simulink model "deadlock"  (Simulink 10.0)
settings: Solver=ode45  StartTime=0.0  StopTime=10  FixedStep=1  MaxStep=inf  RelTol=1e-3  EnableMultiTasking=on
InitFcn:
  | EXT_PACKET = 1;
  | ACK_PACKET = 2;
  | RX = 1;
  | TX = 2;
  | COMMS_DELAY = 1;
libraries: simeventsgenerators1 x8, simeventsserver1 x8, simeventsattributes2 x6, simeventssink1 x4, simeventsgates1 x2, simeventsqueue1 x2, simeventsrouting1 x2, simeventstranslate1 x2, simulink x1
settings Model: Creator=The MathWorks Inc.  LastModifiedBy=bhisma
settings DataIOCC: LimitDataPoints=on  SignalLoggingSaveFormat=ModelDataLogs  SaveOutput=off  SaveTime=off
settings OptimizationCC: ExpressionDepthLimit=2147483647  EfficientMapNaN2IntZero=off
settings DebuggingCC: ReadBeforeWriteMsg=DisableAll  WriteAfterWriteMsg=DisableAll  WriteAfterReadMsg=DisableAll  AlgebraicLoopMsg=error  FcnCallInpInsideContextMsg=warning  StateNameClashWarn=warning
settings SFSimCC: SimParseCustomCode=off
settings GRTTargetCC: GeneratePreprocessorConditionals=Disable all
settings ConfigComp: CovExternalEMLEnable=off
settings SimEventsCC: propDiagAttribOutput=1  propDiagFcnCallOutput=1  propDiagStatOutput=0  propPreventDuplicateEvents=0

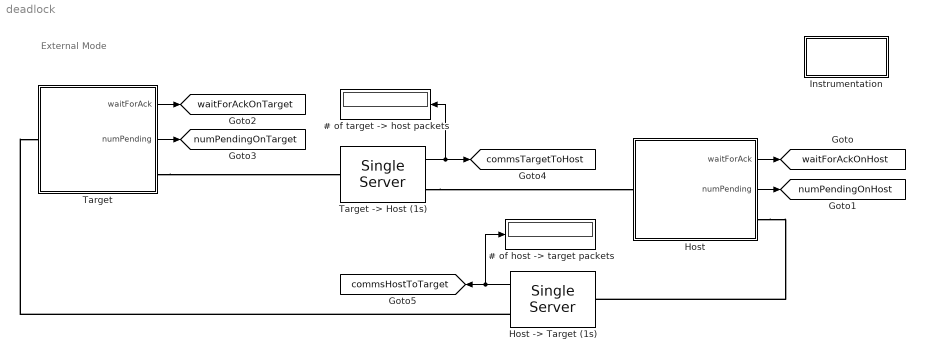
== system deadlock ==
  note: External Mode
  "# of host -> target packets" : Display
  "# of target -> host packets" : Display
  Host : Subsystem
  "Host -> Target (1s)" : simeventsserver1/Single Server  Priority=1  SystemSampleTime=-1  ServiceTimeFrom=Dialog  ServiceTime=COMMS_DELAY  AttributeName=ServiceTime  PriorityServiceCompletion=1  PermitPreemption=off  SortingAttributeName=PriorityAttributeName  SortingDirection=Ascending  WriteToAttribute=off  ResidualAttributeName=ResidualServiceTime  CreateAttribute=on  EnableTOPort=off  StatNumberDeparted=On  StatNumberInBlock=Off  StatNumberPreempted=Off  StatPendingEntity=Off  StatAverageWait=Off  StatUtilization=Off  StatNumberTimedout=Off
  Instrumentation : Subsystem
      settings: RequestExecContextInheritance=on
      mask Display: disp('Scopes');
  Target : Subsystem
  "Target -> Host (1s)" : simeventsserver1/Single Server  Priority=1  SystemSampleTime=-1  ServiceTimeFrom=Dialog  ServiceTime=COMMS_DELAY  AttributeName=ServiceTime  PriorityServiceCompletion=1  PermitPreemption=off  SortingAttributeName=PriorityAttributeName  SortingDirection=Ascending  WriteToAttribute=off  ResidualAttributeName=ResidualServiceTime  CreateAttribute=on  EnableTOPort=off  StatNumberDeparted=On  StatNumberInBlock=Off  StatNumberPreempted=Off  StatPendingEntity=Off  StatAverageWait=Off  StatUtilization=Off  StatNumberTimedout=Off
  tag scope: commsHostToTarget=global, commsTargetToHost=global, numPendingOnHost=global, numPendingOnTarget=global, waitForAckOnHost=global, waitForAckOnTarget=global
  wires:
  Host/1(waitForAck) -> [waitForAckOnHost]
  Host/2(numPending) -> [numPendingOnHost]
  Target/1(waitForAck) -> [waitForAckOnTarget]
  Target/2(numPending) -> [numPendingOnTarget]
  "Target -> Host (1s)"/1 -> [commsTargetToHost], "# of target -> host packets"/1
  "Host -> Target (1s)"/1 -> [commsHostToTarget], "# of host -> target packets"/1
  connections:
  Target/RConn1 -- "Target -> Host (1s)"/LConn1
  "Target -> Host (1s)"/RConn1 -- Host/LConn1
  Host/RConn1 -- "Host -> Target (1s)"/LConn1
  "Host -> Target (1s)"/RConn1 -- Target/LConn1

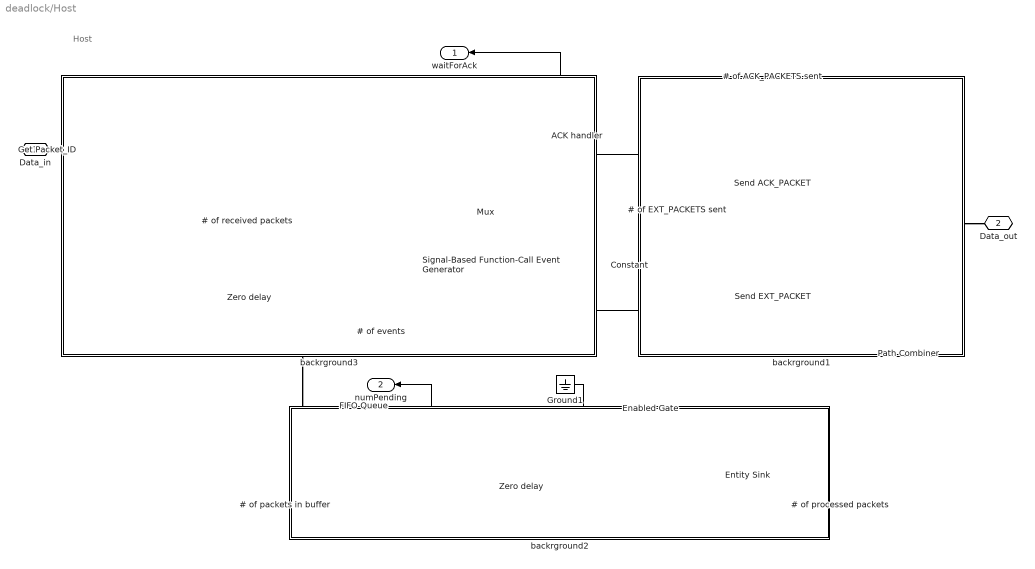
== system deadlock/Host ==
  note: Host
  # of ACK_PACKETS sent : Display
  # of EXT_PACKETS sent : Display
  # of events : Display
  # of packets in buffer : Display
  # of processed packets : Display
  # of received packets : Display
  ACK handler : Stateflow chart  TreatAsAtomicUnit=on
      settings: PropExecContextOutsideSubsystem=on
  Constant : Constant
  Enabled Gate : simeventsgates1/Enabled Gate  Priority=1  SystemSampleTime=-1  SpecifyEventPriority=off  PriorityGateEnableOpenClose=2000  StatNumberDeparted=Off
  Entity Sink : simeventssink1/Entity Sink  Priority=1  SystemSampleTime=-1  AvailableForArrivals=on  StatNumberArrived=On
  FIFO Queue : simeventsqueue1/FIFO Queue  Priority=1  SystemSampleTime=-1  Capacity=2  EnableTOPort=off  StatNumberDeparted=Off  StatNumberInBlock=On  StatPendingEntity=Off  StatAverageWait=Off  StatAverageQueueLength=Off  StatNumberTimedout=Off
      settings: AttributesFormatString=Capacity = %<Capacity>
  Get Packet_ID : simeventsattributes2/Get Attribute  Priority=1  SystemSampleTime=-1  AttributeName=PacketID  AttributeMissing=Error  AttributeDefaultValue=1  AttributeSendTiming=After entity departure  AttributeTreatAsVector=1  StatNumberDeparted=Off  EvaluatedDefaultAttributeValue={[]}
  Ground1 : Ground
  Mux : Mux  Inputs=2
  Path Combiner : simeventsrouting1/Path Combiner  Priority=1  SystemSampleTime=-1  NumberInputPorts=2  InputPortPrecedence=IN1 port  InitialSeed=45675  SpecifyEventPriority=off  PriorityPathCombinerPortPrecedenceSelection=4100  StatNumberDeparted=Off  StatLastArrivalPort=Off  EvaluatedNumPorts=2
  Send ACK_PACKET : Subsystem
  Send EXT_PACKET : Subsystem
  Signal-Based Function-Call Event Generator : simeventsgenerators1/Event Generators/Signal-Based Function-Call Event Generator  Priority=1  SystemSampleTime=-1  GenerateFunctionCallUpon=Change in signal from port vc  SignalEdgeOption=Either  EnableE1Port=off  EnableF2Port=off  EnableE2Port=off  SpecifyEventPriority=off  PriorityFunctionCall=200  FunctionCallDelayFrom=Dialog  DelayFunctionCall=0  StatNumberF1Calls=On  StatNumberF2Calls=Off  MaskBlockType=none
  Zero delay : simeventsserver1/Single Server  Priority=1  SystemSampleTime=-1  ServiceTimeFrom=Dialog  ServiceTime=0  AttributeName=ServiceTime  PriorityServiceCompletion=1  PermitPreemption=off  SortingAttributeName=PriorityAttributeName  SortingDirection=Ascending  WriteToAttribute=off  ResidualAttributeName=ResidualServiceTime  CreateAttribute=on  EnableTOPort=off  StatNumberDeparted=Off  StatNumberInBlock=Off  StatNumberPreempted=Off  StatPendingEntity=Off  StatAverageWait=Off  StatUtilization=Off  StatNumberTimedout=Off
  "Zero delay " : simeventsserver1/Single Server  Priority=1  SystemSampleTime=-1  ServiceTimeFrom=Dialog  ServiceTime=0  AttributeName=ServiceTime  PriorityServiceCompletion=1  PermitPreemption=off  SortingAttributeName=PriorityAttributeName  SortingDirection=Ascending  WriteToAttribute=off  ResidualAttributeName=ResidualServiceTime  CreateAttribute=on  EnableTOPort=off  StatNumberDeparted=On  StatNumberInBlock=On  StatNumberPreempted=Off  StatPendingEntity=Off  StatAverageWait=Off  StatUtilization=Off  StatNumberTimedout=Off
  backrground1 : Subsystem
      mask Display: disp('')
  backrground2 : Subsystem
      mask Display: disp('')
  backrground3 : Subsystem
      mask Display: disp('')
  Data_in : PMIOPort  Side=Left
  Data_out : PMIOPort  Port=2  Side=Right
  waitForAck : Outport
  numPending : Outport  Port=2
  wires:
  Entity Sink/1 -> # of processed packets/1
  Constant/1 -> Send EXT_PACKET/1(waitForAck)
  FIFO Queue/1 -> numPending/1, # of packets in buffer/1
  Get Packet_ID/1 -> ACK handler/1(pID)
  "Zero delay "/2 -> Signal-Based Function-Call Event Generator/1
  ACK handler/1(waitForAck) -> waitForAck/1
  Send ACK_PACKET/1(numAckPacketsSent) -> # of ACK_PACKETS sent/1
  Send EXT_PACKET/1(numExtPacketsSent) -> # of EXT_PACKETS sent/1
  Signal-Based Function-Call Event Generator/2 -> # of events/1
  Mux/1 -> ACK handler/Trigger
  Signal-Based Function-Call Event Generator/1 -> Mux/1
  ACK handler/2(sendAck()) -> Send ACK_PACKET/1(trig)
  Ground1/1 -> Enabled Gate/1
  Send EXT_PACKET/2(txExtPacket) -> Mux/2
  "Zero delay "/1 -> # of received packets/1
  connections:
  Enabled Gate/RConn1 -- Entity Sink/LConn1
  Path Combiner/RConn1 -- Data_out/RConn1
  Send ACK_PACKET/RConn1 -- Path Combiner/LConn1
  Send EXT_PACKET/RConn1 -- Path Combiner/LConn2
  FIFO Queue/RConn1 -- Zero delay/LConn1
  Zero delay/RConn1 -- Enabled Gate/LConn1
  Data_in/RConn1 -- Get Packet_ID/LConn1
  Get Packet_ID/RConn1 -- "Zero delay "/LConn1
  "Zero delay "/RConn1 -- FIFO Queue/LConn1

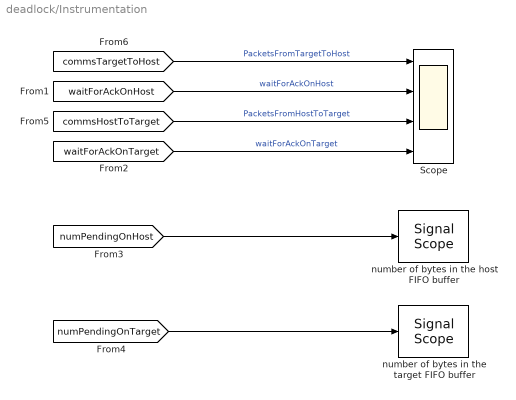
== system deadlock/Instrumentation ==
  Scope : Scope  NumInputPorts=4
  number of bytes in the host FIFO buffer : simeventssink1/Signal Scope  Priority=1  SystemSampleTime=-1  PlotType=Stair  InputType=Signal  NumInputs=1  AttributeNameY=Count  XInputOptionSignal=Event time  XInputOptionEntity=Event time  AttributeNameX=Count  EnableEntityOutport=on  XMin=0  XMax=10  XLimitExceededOption=Stretch axis limits  YLimitExceededOption=Stretch axis limits  AxisGrid=on  AxisLegend=off  LineDisables=""  LineColors=b  LineStyles=-  LineMarkers=.  OpenScopeAtSimStart=on  Title=Packets in host buffer  YLabel=#n  XLabel=Time  FigurePosition=[72 229 231 135]  AxisZoom=off  DataStoreOption=Limited  DataPointsLimit=10000  StatNumberArrived=Off  ShowCountPlotted=off  ShowToolbar=on
      settings: YMin=-1  YMax=3
  number of bytes in the target FIFO buffer : simeventssink1/Signal Scope  Priority=1  SystemSampleTime=-1  PlotType=Stair  InputType=Signal  NumInputs=1  AttributeNameY=Count  XInputOptionSignal=Event time  XInputOptionEntity=Event time  AttributeNameX=Count  EnableEntityOutport=on  XMin=0  XMax=10  XLimitExceededOption=Stretch axis limits  YLimitExceededOption=Stretch axis limits  AxisGrid=on  AxisLegend=off  LineDisables=""  LineColors=b  LineStyles=-  LineMarkers=.  OpenScopeAtSimStart=on  Title=Packets in target buffer  YLabel=#n  XLabel=Time  FigurePosition=[72 229 231 135]  AxisZoom=off  DataStoreOption=Limited  DataPointsLimit=10000  StatNumberArrived=Off  ShowCountPlotted=off  ShowToolbar=on
      settings: YMin=-1  YMax=3
  wires:
  [numPendingOnHost] -> number of bytes in the host FIFO buffer/1
  [numPendingOnTarget] -> number of bytes in the target FIFO buffer/1
  [commsTargetToHost] -> Scope/1  "PacketsFromTargetToHost"
  [waitForAckOnHost] -> Scope/2  "waitForAckOnHost"
  [commsHostToTarget] -> Scope/3  "PacketsFromHostToTarget"
  [waitForAckOnTarget] -> Scope/4  "waitForAckOnTarget"

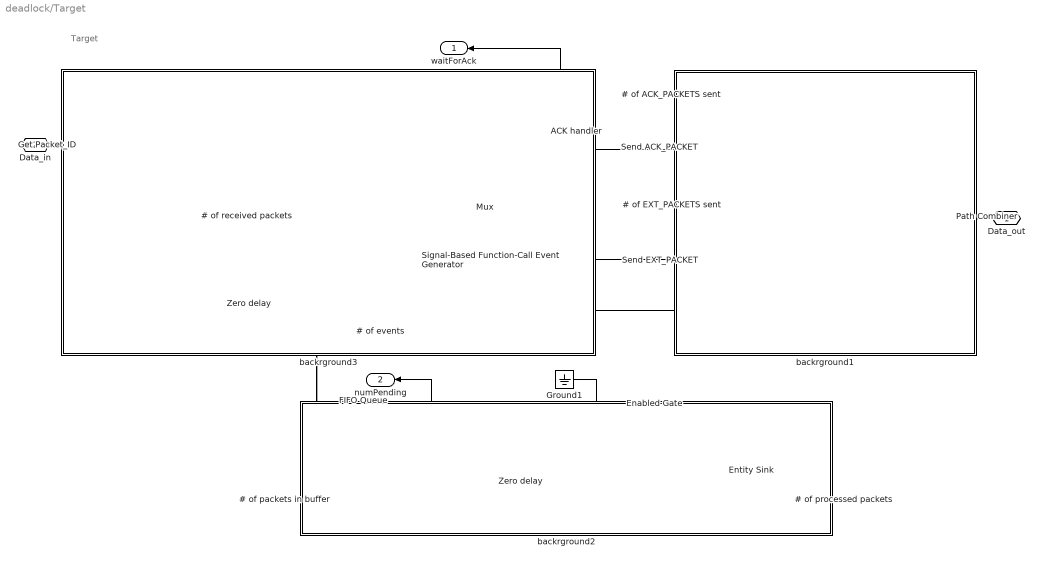
== system deadlock/Target ==
  note: Target
  # of ACK_PACKETS sent : Display
  # of EXT_PACKETS sent : Display
  # of events : Display
  # of packets in buffer : Display
  # of processed packets : Display
  # of received packets : Display
  ACK handler : Stateflow chart  TreatAsAtomicUnit=on
      settings: PropExecContextOutsideSubsystem=on
  Enabled Gate : simeventsgates1/Enabled Gate  Priority=1  SystemSampleTime=-1  SpecifyEventPriority=off  PriorityGateEnableOpenClose=2000  StatNumberDeparted=Off
  Entity Sink : simeventssink1/Entity Sink  Priority=1  SystemSampleTime=-1  AvailableForArrivals=on  StatNumberArrived=On
  FIFO Queue : simeventsqueue1/FIFO Queue  Priority=1  SystemSampleTime=-1  Capacity=2  EnableTOPort=off  StatNumberDeparted=Off  StatNumberInBlock=On  StatPendingEntity=Off  StatAverageWait=Off  StatAverageQueueLength=Off  StatNumberTimedout=Off
      settings: AttributesFormatString=Capacity = %<Capacity>
  Get Packet_ID : simeventsattributes2/Get Attribute  Priority=1  SystemSampleTime=-1  AttributeName=PacketID  AttributeMissing=Error  AttributeDefaultValue=1  AttributeSendTiming=After entity departure  AttributeTreatAsVector=1  StatNumberDeparted=Off  EvaluatedDefaultAttributeValue={[]}
  Ground1 : Ground
  Mux : Mux  Inputs=2
  Path Combiner : simeventsrouting1/Path Combiner  Priority=1  SystemSampleTime=-1  NumberInputPorts=2  InputPortPrecedence=IN1 port  InitialSeed=45675  SpecifyEventPriority=off  PriorityPathCombinerPortPrecedenceSelection=4100  StatNumberDeparted=Off  StatLastArrivalPort=Off  EvaluatedNumPorts=2
  Send ACK_PACKET : Subsystem
  Send EXT_PACKET : Subsystem
  Signal-Based Function-Call Event Generator : simeventsgenerators1/Event Generators/Signal-Based Function-Call Event Generator  Priority=1  SystemSampleTime=-1  GenerateFunctionCallUpon=Change in signal from port vc  SignalEdgeOption=Rising  EnableE1Port=off  EnableF2Port=off  EnableE2Port=off  SpecifyEventPriority=on  PriorityFunctionCall=2  FunctionCallDelayFrom=Dialog  DelayFunctionCall=0  StatNumberF1Calls=On  StatNumberF2Calls=Off  MaskBlockType=none
  Zero delay : simeventsserver1/Single Server  Priority=1  SystemSampleTime=-1  ServiceTimeFrom=Dialog  ServiceTime=0  AttributeName=ServiceTime  PriorityServiceCompletion=1  PermitPreemption=off  SortingAttributeName=PriorityAttributeName  SortingDirection=Ascending  WriteToAttribute=off  ResidualAttributeName=ResidualServiceTime  CreateAttribute=on  EnableTOPort=off  StatNumberDeparted=Off  StatNumberInBlock=Off  StatNumberPreempted=Off  StatPendingEntity=Off  StatAverageWait=Off  StatUtilization=Off  StatNumberTimedout=Off
  "Zero delay " : simeventsserver1/Single Server  Priority=1  SystemSampleTime=-1  ServiceTimeFrom=Dialog  ServiceTime=0  AttributeName=ServiceTime  PriorityServiceCompletion=1  PermitPreemption=off  SortingAttributeName=PriorityAttributeName  SortingDirection=Ascending  WriteToAttribute=off  ResidualAttributeName=ResidualServiceTime  CreateAttribute=on  EnableTOPort=off  StatNumberDeparted=On  StatNumberInBlock=Off  StatNumberPreempted=Off  StatPendingEntity=Off  StatAverageWait=Off  StatUtilization=Off  StatNumberTimedout=Off
  backrground1 : Subsystem
      mask Display: disp('')
  backrground2 : Subsystem
      mask Display: disp('')
  backrground3 : Subsystem
      mask Display: disp('')
  Data_out : PMIOPort  Side=Right
  Data_in : PMIOPort  Port=2  Side=Left
  waitForAck : Outport
  numPending : Outport  Port=2
  wires:
  Send ACK_PACKET/1(numAckPacketsSent) -> # of ACK_PACKETS sent/1
  Send EXT_PACKET/1(numExtPacketsSent) -> # of EXT_PACKETS sent/1
  FIFO Queue/1 -> numPending/1, # of packets in buffer/1
  Get Packet_ID/1 -> ACK handler/1(pID)
  ACK handler/1(waitForAck) -> waitForAck/1, Send EXT_PACKET/1(waitForAck)
  Signal-Based Function-Call Event Generator/2 -> # of events/1
  "Zero delay "/1 -> # of received packets/1, Signal-Based Function-Call Event Generator/1
  Mux/1 -> ACK handler/Trigger
  Signal-Based Function-Call Event Generator/1 -> Mux/1
  ACK handler/2(sendAck()) -> Send ACK_PACKET/1(trig)
  Ground1/1 -> Enabled Gate/1
  Entity Sink/1 -> # of processed packets/1
  Send EXT_PACKET/2(txExtPacket) -> Mux/2
  connections:
  Send ACK_PACKET/RConn1 -- Path Combiner/LConn1
  Send EXT_PACKET/RConn1 -- Path Combiner/LConn2
  Path Combiner/RConn1 -- Data_out/RConn1
  "Zero delay "/RConn1 -- FIFO Queue/LConn1
  FIFO Queue/RConn1 -- Zero delay/LConn1
  Zero delay/RConn1 -- Enabled Gate/LConn1
  Get Packet_ID/RConn1 -- "Zero delay "/LConn1
  Data_in/RConn1 -- Get Packet_ID/LConn1
  Enabled Gate/RConn1 -- Entity Sink/LConn1

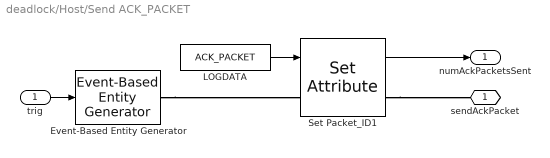
== system deadlock/Host/Send ACK_PACKET ==
  trig : Inport
  Event-Based Entity Generator : simeventsgenerators1/Entity Generators/Event-Based Entity Generator  Priority=1  SystemSampleTime=-1  GenerateEntitiesUpon=Function call from port fcn  SignalEdgeType=Rising  SpecifyEventPriority=off  PriorityEntityGeneration=300  GenerateEntityAtSimulationStart=on  AllowBlocking=on  ResponseDuringBlockage=Delay first pending entity  EntityType=Blank  StatNumberDeparted=Off  StatPendingEntity=Off  StatAverageIntergenerationTime=Off
  LOGDATA : Constant  Value=ACK_PACKET
  Set Packet_ID1 : simeventsattributes2/Set Attribute  Priority=1  SystemSampleTime=-1  AttributeFrom=Signal port  AttributeName=PacketID  AttributeTreatAsVector=1  AttributeValue=1  AttributeCreate=on  StatNumberDeparted=On  EvaluatedAttributeValue={[]}
  sendAckPacket : PMIOPort  Side=Right
  numAckPacketsSent : Outport
  wires:
  LOGDATA/1 -> Set Packet_ID1/1
  trig/1 -> Event-Based Entity Generator/1
  Set Packet_ID1/1 -> numAckPacketsSent/1
  connections:
  Event-Based Entity Generator/RConn1 -- Set Packet_ID1/LConn1
  Set Packet_ID1/RConn1 -- sendAckPacket/RConn1

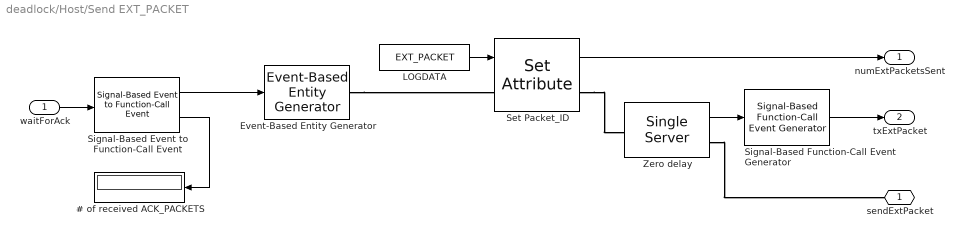
== system deadlock/Host/Send EXT_PACKET ==
  waitForAck : Inport
  # of received ACK_PACKETS : Display
  Event-Based Entity Generator : simeventsgenerators1/Entity Generators/Event-Based Entity Generator  Priority=1  SystemSampleTime=-1  GenerateEntitiesUpon=Function call from port fcn  SignalEdgeType=Falling  SpecifyEventPriority=off  PriorityEntityGeneration=300  GenerateEntityAtSimulationStart=on  AllowBlocking=on  ResponseDuringBlockage=Delay first pending entity  EntityType=Blank  StatNumberDeparted=Off  StatPendingEntity=Off  StatAverageIntergenerationTime=Off
  LOGDATA : Constant  Value=EXT_PACKET
  Set Packet_ID : simeventsattributes2/Set Attribute  Priority=1  SystemSampleTime=-1  AttributeFrom=Signal port  AttributeName=PacketID  AttributeTreatAsVector=1  AttributeValue=1  AttributeCreate=on  StatNumberDeparted=On  EvaluatedAttributeValue={[]}
  Signal-Based Function-Call Event Generator : simeventsgenerators1/Event Generators/Signal-Based Function-Call Event Generator  Priority=1  SystemSampleTime=-1  GenerateFunctionCallUpon=Change in signal from port vc  SignalEdgeOption=Either  EnableE1Port=off  EnableF2Port=off  EnableE2Port=off  SpecifyEventPriority=off  PriorityFunctionCall=200  FunctionCallDelayFrom=Dialog  DelayFunctionCall=0  StatNumberF1Calls=Off  StatNumberF2Calls=Off  MaskBlockType=none
  Signal-Based Event to Function-Call Event : simeventstranslate1/Signal-Based Event to Function-Call Event  Priority=1  SystemSampleTime=-1  GenerateFunctionCallUpon=Change in signal from port vc  SignalEdgeOption=Falling  EnableE1Port=off  EnableF2Port=off  EnableE2Port=off  SpecifyEventPriority=off  PriorityFunctionCall=200  FunctionCallDelayFrom=Dialog  DelayFunctionCall=0  StatNumberF1Calls=On  StatNumberF2Calls=Off  MaskBlockType=none
  "Zero delay " : simeventsserver1/Single Server  Priority=1  SystemSampleTime=-1  ServiceTimeFrom=Dialog  ServiceTime=0  AttributeName=ServiceTime  PriorityServiceCompletion=1  PermitPreemption=off  SortingAttributeName=PriorityAttributeName  SortingDirection=Ascending  WriteToAttribute=off  ResidualAttributeName=ResidualServiceTime  CreateAttribute=on  EnableTOPort=off  StatNumberDeparted=Off  StatNumberInBlock=On  StatNumberPreempted=Off  StatPendingEntity=Off  StatAverageWait=Off  StatUtilization=Off  StatNumberTimedout=Off
  sendExtPacket : PMIOPort  Side=Right
  numExtPacketsSent : Outport
  txExtPacket : Outport  Port=2
  wires:
  LOGDATA/1 -> Set Packet_ID/1
  Set Packet_ID/1 -> numExtPacketsSent/1
  Signal-Based Event to Function-Call Event/2 -> # of received ACK_PACKETS/1
  Signal-Based Event to Function-Call Event/1 -> Event-Based Entity Generator/1
  waitForAck/1 -> Signal-Based Event to Function-Call Event/1
  "Zero delay "/1 -> Signal-Based Function-Call Event Generator/1
  Signal-Based Function-Call Event Generator/1 -> txExtPacket/1
  connections:
  Event-Based Entity Generator/RConn1 -- Set Packet_ID/LConn1
  Set Packet_ID/RConn1 -- "Zero delay "/LConn1
  "Zero delay "/RConn1 -- sendExtPacket/RConn1

== system deadlock/Host/backrground1 ==

== system deadlock/Host/backrground2 ==

== system deadlock/Host/backrground3 ==

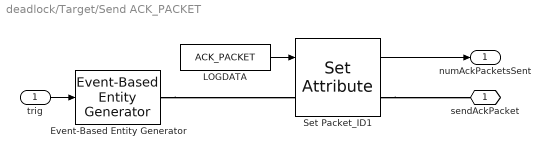
== system deadlock/Target/Send ACK_PACKET ==
  trig : Inport
  Event-Based Entity Generator : simeventsgenerators1/Entity Generators/Event-Based Entity Generator  Priority=1  SystemSampleTime=-1  GenerateEntitiesUpon=Function call from port fcn  SignalEdgeType=Rising  SpecifyEventPriority=off  PriorityEntityGeneration=300  GenerateEntityAtSimulationStart=on  AllowBlocking=on  ResponseDuringBlockage=Delay first pending entity  EntityType=Blank  StatNumberDeparted=Off  StatPendingEntity=Off  StatAverageIntergenerationTime=Off
  LOGDATA : Constant  Value=ACK_PACKET
  Set Packet_ID1 : simeventsattributes2/Set Attribute  Priority=1  SystemSampleTime=-1  AttributeFrom=Signal port  AttributeName=PacketID  AttributeTreatAsVector=1  AttributeValue=1  AttributeCreate=on  StatNumberDeparted=On  EvaluatedAttributeValue={[]}
  sendAckPacket : PMIOPort  Side=Right
  numAckPacketsSent : Outport
  wires:
  LOGDATA/1 -> Set Packet_ID1/1
  trig/1 -> Event-Based Entity Generator/1
  Set Packet_ID1/1 -> numAckPacketsSent/1
  connections:
  Event-Based Entity Generator/RConn1 -- Set Packet_ID1/LConn1
  Set Packet_ID1/RConn1 -- sendAckPacket/RConn1

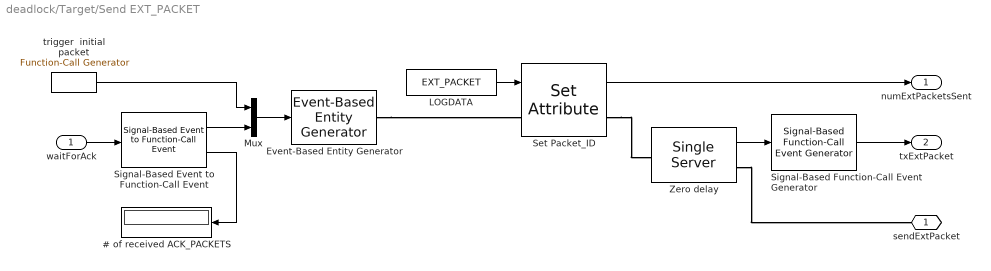
== system deadlock/Target/Send EXT_PACKET ==
  waitForAck : Inport
  # of received ACK_PACKETS : Display
  Event-Based Entity Generator : simeventsgenerators1/Entity Generators/Event-Based Entity Generator  Priority=1  SystemSampleTime=-1  GenerateEntitiesUpon=Function call from port fcn  SignalEdgeType=Falling  SpecifyEventPriority=off  PriorityEntityGeneration=300  GenerateEntityAtSimulationStart=on  AllowBlocking=on  ResponseDuringBlockage=Delay first pending entity  EntityType=Blank  StatNumberDeparted=Off  StatPendingEntity=Off  StatAverageIntergenerationTime=Off
  LOGDATA : Constant  Value=EXT_PACKET
  Mux : Mux  Inputs=2
  Set Packet_ID : simeventsattributes2/Set Attribute  Priority=1  SystemSampleTime=-1  AttributeFrom=Signal port  AttributeName=PacketID  AttributeTreatAsVector=1  AttributeValue=1  AttributeCreate=on  StatNumberDeparted=On  EvaluatedAttributeValue={[]}
  Signal-Based Function-Call Event Generator : simeventsgenerators1/Event Generators/Signal-Based Function-Call Event Generator  Priority=1  SystemSampleTime=-1  GenerateFunctionCallUpon=Change in signal from port vc  SignalEdgeOption=Either  EnableE1Port=off  EnableF2Port=off  EnableE2Port=off  SpecifyEventPriority=off  PriorityFunctionCall=200  FunctionCallDelayFrom=Dialog  DelayFunctionCall=0  StatNumberF1Calls=Off  StatNumberF2Calls=Off  MaskBlockType=none
  Signal-Based Event to Function-Call Event : simeventstranslate1/Signal-Based Event to Function-Call Event  Priority=1  SystemSampleTime=-1  GenerateFunctionCallUpon=Change in signal from port vc  SignalEdgeOption=Falling  EnableE1Port=off  EnableF2Port=off  EnableE2Port=off  SpecifyEventPriority=off  PriorityFunctionCall=200  FunctionCallDelayFrom=Dialog  DelayFunctionCall=0  StatNumberF1Calls=On  StatNumberF2Calls=Off  MaskBlockType=none
  "Zero delay " : simeventsserver1/Single Server  Priority=1  SystemSampleTime=-1  ServiceTimeFrom=Dialog  ServiceTime=0  AttributeName=ServiceTime  PriorityServiceCompletion=1  PermitPreemption=off  SortingAttributeName=PriorityAttributeName  SortingDirection=Ascending  WriteToAttribute=off  ResidualAttributeName=ResidualServiceTime  CreateAttribute=on  EnableTOPort=off  StatNumberDeparted=Off  StatNumberInBlock=On  StatNumberPreempted=Off  StatPendingEntity=Off  StatAverageWait=Off  StatUtilization=Off  StatNumberTimedout=Off
  trigger  initial packet : simulink/Ports & Subsystems/Function-Call Generator  sample_time=1e10  numberOfIterations=1
  sendExtPacket : PMIOPort  Side=Right
  numExtPacketsSent : Outport
  txExtPacket : Outport  Port=2
  wires:
  LOGDATA/1 -> Set Packet_ID/1
  Set Packet_ID/1 -> numExtPacketsSent/1
  trigger  initial packet/1 -> Mux/1
  Signal-Based Event to Function-Call Event/2 -> # of received ACK_PACKETS/1
  Signal-Based Event to Function-Call Event/1 -> Mux/2
  waitForAck/1 -> Signal-Based Event to Function-Call Event/1
  Mux/1 -> Event-Based Entity Generator/1
  "Zero delay "/1 -> Signal-Based Function-Call Event Generator/1
  Signal-Based Function-Call Event Generator/1 -> txExtPacket/1
  connections:
  Event-Based Entity Generator/RConn1 -- Set Packet_ID/LConn1
  Set Packet_ID/RConn1 -- "Zero delay "/LConn1
  "Zero delay "/RConn1 -- sendExtPacket/RConn1

== system deadlock/Target/backrground1 ==

== system deadlock/Target/backrground2 ==

== system deadlock/Target/backrground3 ==

== stateflow chart Target/ACK handler ==
  state default
    % idle
  state waiting
    en: waitForAck = 1;
  state ready
    en: waitForAck = 0;
  ready -> ready [order 1] : rx [pID == EXT_PACKET] {sendAck}
  default -> ready [order 2] : rx [pID == EXT_PACKET] {sendAck}
  ready -> waiting [order 2] : tx
  waiting -> ready [order 1] : rx [pID == ACK_PACKET]
  default -> ready [order 1] : rx [pID == ACK_PACKET]
  default -> waiting [order 3] : tx
  waiting -> waiting [order 2] : rx [pID == EXT_PACKET] {sendAck}
  (default) -> default : {waitForAck = 0;}
  data: waitForAck output double; ACK_PACKET parameter double; EXT_PACKET parameter double; pID input double
  events: sendAck output FUNCTION_CALL_EVENT; rx input FUNCTION_CALL_EVENT; tx input FUNCTION_CALL_EVENT

== stateflow chart Host/ACK handler ==
  state default
    % idle
  state waiting
    en: waitForAck = 1;
  state ready
    en: waitForAck = 0;
  ready -> ready [order 1] : rx [pID == EXT_PACKET] {sendAck;}
  default -> ready [order 2] : rx [pID == EXT_PACKET] {sendAck;}
  ready -> waiting [order 2] : tx
  waiting -> ready [order 1] : rx [pID == ACK_PACKET]
  default -> ready [order 1] : rx [pID == ACK_PACKET]
  default -> waiting [order 3] : tx
  waiting -> waiting [order 2] : rx [pID == EXT_PACKET] {sendAck;}
  (default) -> default : {waitForAck = 0;}
  data: waitForAck output double; ACK_PACKET parameter double; EXT_PACKET parameter double; pID input double
  events: sendAck output FUNCTION_CALL_EVENT; rx input FUNCTION_CALL_EVENT; tx input FUNCTION_CALL_EVENT
